simulink model "Microgrid_transition_model_15July2021"  (R2020a)
settings: Solver=VariableStepAuto  StartTime=0.0  StopTime=10  MaxStep=1e-4  RelTol=1e-3
PreLoadFcn:
  | run('FC_microgrid_param.m')
InitFcn:
  | %load myisoModel_init;
  | run('FC_microgrid_param.m')
  | tic
  | run('CARTinitFcn.m')
  | %caseNo = 2;
  | 
  | %if (caseNo == 1)
  | %set_param(['Isolated_grid_paper_model_022521/SignalGen'], 'ActiveScenario', 'PStep222kW');
  | %else
  | %set_param(['Isolated_grid_paper_model_022521/SignalGen'], 'ActiveScenario', 'QStep222kVAr');
  | 
  | %end;
StopFcn:
  | toc
undefined symbols (not defined in the file): breakpoints1, breakpoints2, cp_table_data, ctrl, D1, Delta, DiscIntNeverNeededParam, DT, FC_BESS, find_system, gcbh, libFC_BESS, oversize, pq_ts, sps_rtmsupport, timer, Ts, ts, Ts_APC, Ts_Control, Ts_Power
libraries: powerlib x107, powerlib_meascontrol x56, powerlib_extras x40, simulink x27, simulink_extras x12, sps_avr x7, pi_ctrl x4, SignalEditorBlockLib x2, libLgBattery x1, libFC_PV x1, eePowerMeasurement x1, spsDieselMotorModel x1
(part 10 of 10)

== matlab function Microgrid_transition_model_15July2021/Wind Turbine Type 2/APC (atomic)/Inertial Response (to df)/TLIC original 1/adaptive TLIC ==
  data: Pmppt input; Delta_P output; Wi input; Act input; S output; Pitch input
function [Delta_P,S]  = TLIC(Pmppt,Wi,Act,Pitch)
%Modified torque-limit based inertial control, originally by Moses
% persistent variables
persistent initFlag; %determine if the varaibles are initialized
persistent Dec_T;
persistent P_last;
persistent P_acc;
persistent W_last;
persistent Index;
persistent W_pre;
persistent Acc;
persistent stages;
persistent T_Stage1;

T_limit=1.1;
W_min=0.5;
Delta_P=0;


if isempty(initFlag) || Act<0.5 
    initFlag = 1; %initialized
    Dec_T =  0;
    P_last = 0;
    P_acc = 0;
    W_last = 0;
    W_pre=0;
    Index=0;
    Acc=0;
    T_Stage1=20;
end

if (Act>=0.5 && Dec_T<T_Stage1)
    stages=1;
elseif (Act>=0.5 && Dec_T>=T_Stage1)
    stages=2;
else
    stages=0;
end

switch stages
    case 0
        Delta_P=0;
        W_pre=Wi;
    case 1
        K_slope=(T_limit*W_pre-W_min^3)/(W_pre-W_min);
        Delta_P=K_slope*(Wi-W_min)+W_min^3-Pmppt;
        P_last=Delta_P+Pmppt;
        W_last=Wi;
        P_acc=P_last;
        Dec_T=Dec_T+0.01;
        if abs(Pitch-0)>1 && Dec_T>=3
            T_Stage1=3;
        end
    case 2
        Index=Index+1;
        % check acceleration
        if Index==(1/2e-6)
            Index=0;
            if Wi-W_last<=0.02
                Acc=1;
            else
                Acc=0;
            end
            W_last=Wi;
        end
        % deloading
        if Acc
            P_acc=P_acc-0.01/100;
        end
        Delta_P=P_acc-Pmppt;
        % terminate inertial
        if Delta_P<=1e-3
            Delta_P=0;
        end
end

S=stages;
        
end

== matlab function Microgrid_transition_model_15July2021/Wind Turbine Type 2/APC (atomic)/Inertial Response (to df)/TLIC2/adaptive TLIC ==
  data: recharge input; trecharge input; tIR input; Delta_P output; Act input; Ts_APC parameter; recharge output; trecharge output; tIR output; tsim input
function [Delta_P, recharge, trecharge, tIR] = TLIC(recharge, trecharge, tIR, Act, Ts_APC, tsim)
%If frequency dips below deadband, provide max torque until rotor
%decelerates to x%. Then resume normal operation

Pmax = 1.3; %max power 1.3 pu

if recharge
    trecharge = trecharge + Ts_APC;
    Delta_P = 0;
    tIR = 0;
    if trecharge > 10
        recharge = 0;
    end
else
    trecharge = 0;
    if Act > 0.5 && tsim >= 10 && tsim < 13
        if tIR <= 3     % was 4 on orginal 
            Delta_P = Pmax-1;
            tIR = tIR + Ts_APC;
        else
            Delta_P = 0;
            tIR = 0;
            recharge = 1;
        end
    else
        Delta_P = 0;
        tIR = 0;
    end
end

== matlab function Microgrid_transition_model_15July2021/Wind Turbine Type 2/Fault Controller (atomic) /turbine_safety  ==
  data: ctrl input Bus: ctrlBus; data input Bus: dataBus; ctrl output; timer input Bus: timerBus; timer output; faulty parameter; dt input
 function [ctrl, timer]   = turbine_safety(ctrl, data, timer, faulty, dt)
    % Fault adaptive controller. Checks various sensor readings, and
    % responds by entering the appropriate control mode, providing the
    % appropriate torque derate, and setting the appropriate timers.
          
    % if faulted, don't change anything 
    if ctrl.mode(4)+ctrl.mode(5)+ctrl.mode(6) == 0 %if not faulted
        ctrl.RP_prev = ctrl.mode(2); %0 if ctrl.cmd =0; 1 otherwise
        fields = fieldnames(faulty); %run warning logic for all faultys
        ctrl.mode = [0,0,0,0,0,0];
        for i=1:length(fields)
            ctrl.(fields{i}).state = 0;
            checkHandle = str2func(faulty.(fields{i}).checkFun); %check for warnings/faultys
            ctrl = checkHandle(data, ctrl);
            ctrl = setMode(ctrl, faulty, fields{i}); %set mode
        end
        [ctrl, timer] = setTimers(ctrl, timer, dt); %set timers and torque derate
        ctrl.modeValue = sum(ctrl.mode.*2.^linspace(0,5,6));
    else
        if ctrl.mode(6) == 1
            fprintf('EMERGENCY STOP')
        elseif ctrl.mode(5) == 1
            fprintf('OPEN LOOP NORMAL STOP')
        elseif ctrl.mode(4) == 1
            fprintf('NORMAL STOP')
        end

%     displays for testing
%         disp('ctrl.mode:')
%         disp(ctrl.mode)
%         disp('data:')
%         disp(data)
%         disp('timer:')
%         disp(timer)
%         fprintf('data = %1.0f\n', data);
%         fprintf('ctrl.Ttarget = %1.0f\n', ctrl.Ttarget);

    end
